simulink model "Lab_2_H036"  (R2022b)
settings: Solver=VariableStepAuto  StartTime=0.0  StopTime=100  RelTol=1e-3
undefined symbols (not defined in the file): B, K, M
settings Model: Creator=abc  LastModifiedBy=abc

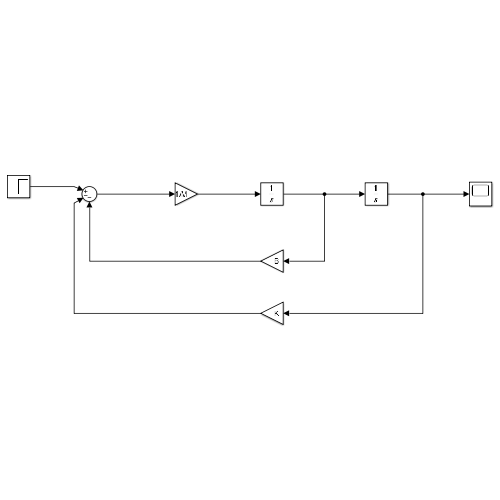
[thumbnail: Simulink's stored preview of the top-level diagram]
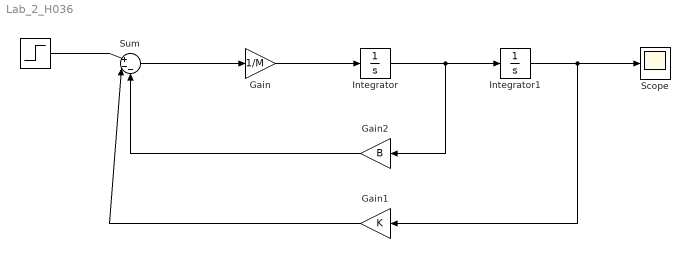
== system Lab_2_H036 ==
  " " : Step  SampleTime=0
  Gain : Gain  Gain=1/M
  Gain1 : Gain  Gain=K
  Gain2 : Gain  Gain=B
  Integrator : Integrator
  Integrator1 : Integrator
  Scope : Scope
  Sum : Sum  Inputs=|+--
  wires:
  Gain/1 -> Integrator/1
  Integrator/1 -> Gain2/1, Integrator1/1
  Integrator1/1 -> Gain1/1, Scope/1
  Gain2/1 -> Sum/3
  Gain1/1 -> Sum/2
  Sum/1 -> Gain/1
  " "/1 -> Sum/1
